simulink model "HEVPlant_Ptbs_V1b_MkSfunc"  (R2018b)
settings: configuration reference "Config_Plant_MkSfunc_FIxStep" (kept outside this file)
PreLoadFcn:
  | HEVPlant_Ptbs_V1_BusInfo
model workspace (MAT data in the model file):
  DiffRatio = 3.421
  EV_current = 200
  EV_motion = [20 4 0.8]
  EV_sf = 2000
  EngDriveRatio = 0.813008130081
  Fs = 0
  Fv = 0.0025
  Jcomp = 0.0227
  Jengine = 0.22
  Ki = 251.3274
  Kisa = 346.6583
  Kp_d = 0.47149
  Kp_q = 0.52125
  Ksa = 85.4316
  Ksf = 1996.2651
  Ld = 0.0003752
  Ldq = [0.0003752 0.0004148]
  Lq = 0.0004148
  Mechanical = [0.0227 0.0025 0]
  MotGbRatio = 1
  P = 4
  PolePairs = 4
  RWheel = 0.3
  Rs = 0.2
  T_max = 120
  T_mtpa = [0 13.3131834767 26.6278836885 39.9456159322 53.2678926341 66.5962219318 79.9321062746 93.277041051 106.632513247 120.000000141]
  b_axle = Simulink.Parameter
  b_axle.Value = 10
  b_axle.DataType = 'auto'
  b_axle.Dimensions = [1 1]
  b_driveshaft = Simulink.Parameter
  b_driveshaft.Value = 10
  b_driveshaft.DataType = 'auto'
  b_driveshaft.Dimensions = [1 1]
  ba = 3.4029
  id_mtpa = [0 -0.114523352646 -0.457989076459 -1.03008464374 -1.83029075221 -2.85788367342 -4.11193850568 -5.59133329791 -7.29475400168 -9.22070020138]
  idq0 = [0 0]
  idq_limits = [-9.220699542 166.993501392 167.247872355]
  iq_mtpa = [0 18.5827440345 37.1633719111 55.7397734896 74.3098506185 92.871523015 111.422734008 129.961456105 148.485696337 166.993501356]
  k_axle = Simulink.Parameter
  k_axle.Value = 5000
  k_axle.DataType = 'auto'
  k_axle.Dimensions = [1 1]
  k_driveshaft = Simulink.Parameter
  k_driveshaft.Value = 1000
  k_driveshaft.DataType = 'auto'
  k_driveshaft.Dimensions = [1 1]
  lambda_pm = 0.1194
  mechanical = [0.0227 0.0025 0]
  mot.max_trq = 307
  mot.max_pwr = 124
  mot.spd = [0 500 1000 1500 2000 2500 3000 3500 3857.04487493 4000 4500 5000 5500 6000 6500 7000 7500 8000 8500 9000 9500 10000 10500 11000 11500 12000 12500]
  mot.trq = [307 307 307 307 307 307 307 307 307 296.028194151 263.136172579 236.822555321 215.29323211 197.352129434 182.171196401 169.158968086 157.881703547 148.014097075 139.307385483 131.568086289 124.643450169 118.41127766 112.772645391 107.646616055 102.9663284 98.676064717 94.7290221283]
  mot.trq_cp = [296.028194151 263.136172579 236.822555321 215.29323211 197.352129434 182.171196401 169.158968086 157.881703547 148.014097075 139.307385483 131.568086289 124.643450169 118.41127766 112.772645391 107.646616055 102.9663284 98.676064717 94.7290221283]
  mot.J = 0.02
  mot.damp = 0.0001
  mot.Tc = 0.0267
  mot.map.spdindex = [0 1000 2000 3000 3857 4000 5000 6000 7000 8000 9000 10000 11000 12000 12584]
  mot.map.trqindex = [10 25 50 75 100 125 150 175 200 225 250 275 300 307]
  mot.map.eff = [84  90  90  90  90  90  90  90  90  90  90  90  90  90  90; 84  90  93  95  95  95  96  95  95  95  95  93  93  93  93; 84  90  93  95  95  95  96  95  96  95  95  95  95  93  93; 84  90  93  95  95  95  96  96  96  95  95  95  95  93  93; 84  90  93  95  95  95  96  96  96  95  95  93  93  93  90; 84  88  90  93  93  95  95  96  95  95  95  93  93  93  90; 84  88  90  90  90  93  95  95  95  93  93  93  93  93  90; 84  88  90  90  90  90  93  93  93  93  93  93  93  93  90; 84  84  88  90  90  90  93  93  93  93  93  93  93  93  90; 84  84  88  90  90  90  90  93  93  93  93  93  93  93  90; 84  84  84  90  90  90  90  93  93  93  93  93  93  93  90; 84  84  84  88  90  90  90  93  93  93  93  93  93  93  90; 84  84  84  88  88  88  90  93  93  93  93  93  93  93  90; 84  84  84  88  88  88  90  93  93  93  93  93  93  93  90]
  mot.m = 30
  mot.Cp = 200
  omega_init = 0
  theta_init = 0
  wc_shaft = Simulink.Parameter
  wc_shaft.Value = 0.1
  wc_shaft.DataType = 'auto'
  wc_shaft.Dimensions = [1 1]
libraries: autolibshared x4, autolibsharedcoupling x2, autolibtransamt x1, autolibshareddiff x1, autolibsharedmappedengines x1, simulink x1, autolibdatasheetbattery x1, autolibmappedmotor x1
(part 1 of 5)
settings Model: Creator=IAEC Nishito  LastModifiedBy=E00026
settings ConfigSetRef: SourceLocation=Base Workspace

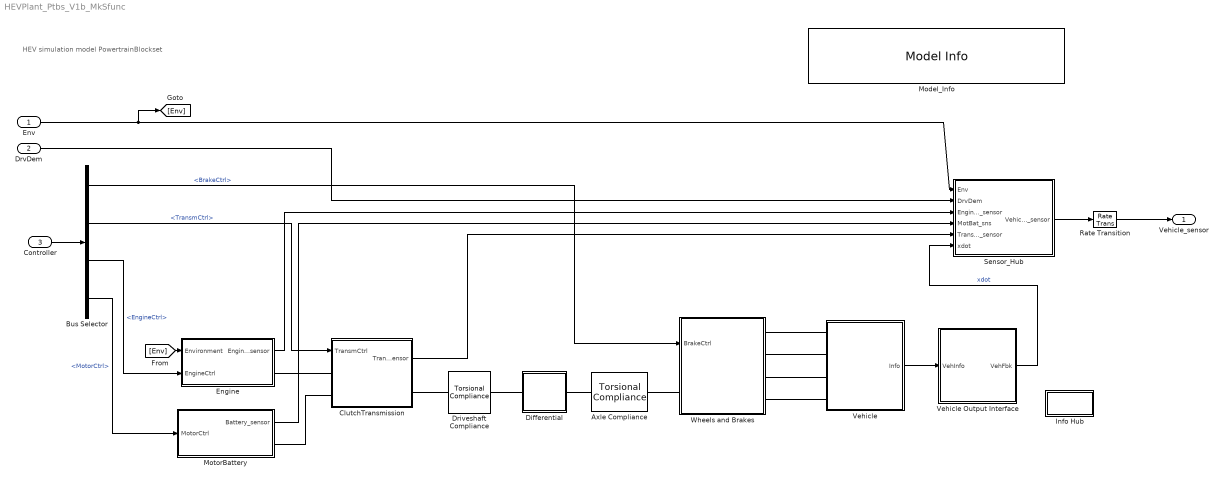
== system HEVPlant_Ptbs_V1b_MkSfunc ==
  note: HEV simulation model
      | PowertrainBlockset
  Env : Inport  OutDataTypeStr=Bus: Environment_Bus  SampleTime=0.001
  DrvDem : Inport  Port=2  OutDataTypeStr=Bus: Driver_demand_Bus  SampleTime=0.001
  Controller : Inport  Port=3  OutDataTypeStr=Bus: Ctrl_intg_Bus  SampleTime=0.001
      settings: AttributesFormatString=%<OutDataTypeStr>
  Axle Compliance : autolibsharedcoupling/Torsional Compliance  port_config=Two-way connection  k=k_axle  b=b_axle  theta_o=0  domega_o=0  omega_c=wc_shaft  blkID=0  aMode=1
      settings: SourceProductName=Powertrain Blockset  SourceProductBaseCode=PW
  Bus Selector : BusSelector  OutputSignals=BrakeCtrl,TransmCtrl,EngineCtrl,MotorCtrl
  ClutchTransmission : Subsystem
  Differential : Subsystem
  Driveshaft Compliance : autolibsharedcoupling/Torsional Compliance  port_config=Two-way connection  k=k_driveshaft  b=b_driveshaft  theta_o=0  domega_o=0  omega_c=wc_shaft  blkID=0  aMode=1
      settings: SourceProductName=Powertrain Blockset  SourceProductBaseCode=PW
  Engine : Subsystem
  Info Hub : Subsystem
  Model_Info : simulink/Model-Wide Utilities/Model Info  Frame=on  DisplayStringWithTags=|  HorizontalTextAlignment=Left  LeftAlignmentValue=0.02
      | Version  %<ModelVersion>
      | LastModifided by %<LastModifiedBy>  Date %<LastModificationDate>
      | Description  %<Description>
  MotorBattery : Subsystem
  Rate Transition : RateTransition  Deterministic=off
  Sensor_Hub : Subsystem
  Vehicle : Subsystem
  Vehicle Output Interface : Subsystem
  Wheels and Brakes : Subsystem
  Vehicle_sensor : Outport  OutDataTypeStr=Bus: Vehicle_sensor_Bus
      settings: AttributesFormatString=%<OutDataTypeStr>
  wires:
  Sensor_Hub/1(Vehicle_sensor) -> Rate Transition/1
  MotorBattery/1(Battery_sensor) -> Sensor_Hub/4(MotBat_sns)
  Env/1 -> [Env], Sensor_Hub/1(Env)
  Bus Selector/3 -> Engine/2(EngineCtrl)  "<EngineCtrl>"
  Bus Selector/1 -> Wheels and Brakes/1(BrakeCtrl)  "<BrakeCtrl>"
  [Env] -> Engine/1(Environment)
  Engine/1(Engine_sensor) -> Sensor_Hub/3(Engine_sensor)
  DrvDem/1 -> Sensor_Hub/2(DrvDem)
  Bus Selector/4 -> MotorBattery/1(MotorCtrl)  "<MotorCtrl>"
  Vehicle Output Interface/1(VehFbk) -> Sensor_Hub/6(xdot)  "xdot"
  Vehicle/1(Info) -> Vehicle Output Interface/1(VehInfo)
  Controller/1 -> Bus Selector/1
  ClutchTransmission/1(Transm_sensor) -> Sensor_Hub/5(Transm_sensor)
  Bus Selector/2 -> ClutchTransmission/1(TransmCtrl)  "<TransmCtrl>"
  Rate Transition/1 -> Vehicle_sensor/1
  connections:
  Driveshaft Compliance/RConn1 -- Differential/LConn1
  Driveshaft Compliance/LConn1 -- ClutchTransmission/RConn1
  Engine/RConn1 -- ClutchTransmission/LConn1
  Wheels and Brakes/RConn2 -- Vehicle/LConn2
  Axle Compliance/LConn1 -- Differential/RConn1
  MotorBattery/RConn1 -- ClutchTransmission/LConn2
  Vehicle/LConn1 -- Wheels and Brakes/RConn1
  Wheels and Brakes/RConn3 -- Vehicle/LConn3
  Axle Compliance/RConn1 -- Wheels and Brakes/LConn1
  Wheels and Brakes/RConn4 -- Vehicle/LConn4

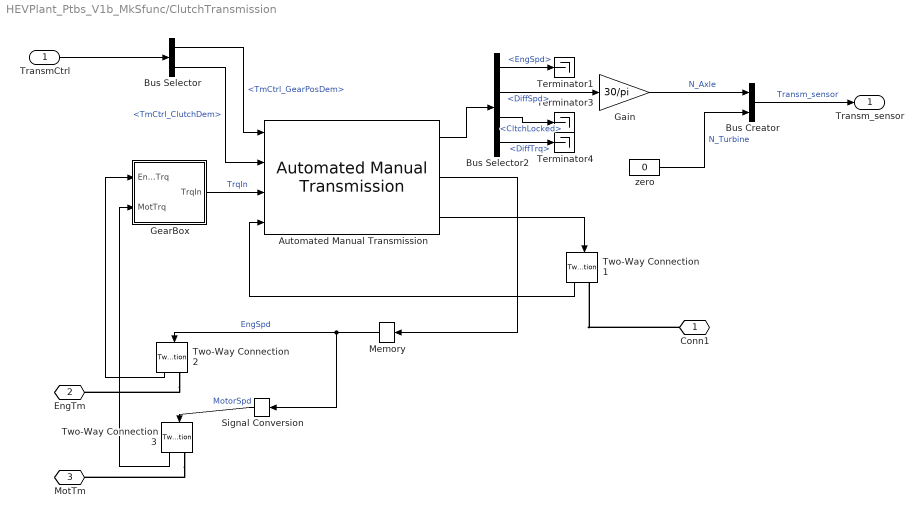
== system HEVPlant_Ptbs_V1b_MkSfunc/ClutchTransmission ==
  TransmCtrl : Inport
  Automated Manual Transmission : autolibtransamt/Automated Manual Transmission  VariantControl=0  cntrlType=External control  TransEffModelPopup=Gear only  Jin=.3  bin=.03  omegain_o=0  G=[-1, 0, 1, 2, 3, 4, 5]  Trq_bpts=[25, 50, 75, 100, 150, 200, 250]  omega_bpts=[52.4 78.5 105 131 157 183 209 262 314 419 524]  Temp_bpts=[313 358]  N=[-4.47 ,1, 4.47, 2.47, 1.47, 1, 0.8]  Jout=[0.128 0.01 0.128 0.1 0.062 0.028 0.01]  bout=[.003 .001 .003 .0025 .002 .001 .001]  eta=[0.9, 0.9, 0.9, 0.9, 0.9, 0.95, 0.95]  eta_tbl=reshape([0.53 0.71 0.77 0.79 0.82 0.82 0.82 0.5 0.7 0.77 0.79 0.82 0.82 0.82 0.54 0.72 0.78 0.81 0.83 0.82 0.82 0.56 0.73 0.79 0.81 0.84 0.82 0.82 0.58 0.74 0.79 0.82 0.84 0.82 0.82 0.57 0.74 0.79 0.82 0.84 0.82 0.82 0.58 0.74 0.79 0.82 0.84 0.82 0.82 0.58 0.74 0.79 0.82 0.84 0.82 0.82 0.57 0.74 0.8 0.82 0.85 0.82 0.82 0.55 0.73 0.78 0.81 0.84 0.82 0.82 0.51 0.71 0.77 0.81 0.84 0.82 0.82 0.53 0.71 0.77 0.79 0.82 0.82 0.82 0.5 0.7 0.77 0.79 0.82 0.82 0.82 0.54 0.72 0.78 0.81 0.83 0.82 0.82 0.56 0.73 0.79 0.81 0.84 0.82 0.82 0.58 0.74 0.79 0.82 0.84 0.82 0.82 0.57 0.74 0.79 0.82 0.84 0.82 0.82 0.58 0.74 0.79 0.82 0.84 0.82 0.82 0.58 0.74 0.79 0.82 0.84 0.82 0.82 0.57 0.74 0.8 0.82 0.85 0.82 0.82 0.55 0.73 0.78 0.81 0.84 0.82 0.82 0.51 0.71 0.77 0.81 0.84 0.82 0.82 0.53 0.71 0.77 0.79 0.82 0.82 0.82 0.5 0.7 0.77 0.79 0.82 0.82 0.82 0.54 0.72 0.78 0.81 0.83 0.82 0.82 0.56 0.73 0.79 0.81 0.84 0.82 0.82 0.58 0.74 0.79 0.82 0.84 0.82 0.82 0.57 0.74 0.79 0.82 0.84 0.82 0.82 0.58 0.74 0.79 0.82 0.84 0.82 0.82 0.58 0.74 0.79 0.82 0.84 0.82 0.82 0.57 0.74 0.8 0.82 0.85 0.82 0.82 0.55 0.73 0.78 0.81 0.84 0.82 0.82 0.51 0.71 0.77 0.81 0.84 0.82 0.82 0.7 0.79 0.82 0.83 0.84 0.84 0.84 0.63 0.76 0.8 0.82 0.83 0.84 0.84 0.58 0.74 0.79 0.81 0.83 0.84 0.84 0.58 0.74 0.79 0.81 0.83 0.84 0.84 0.58 0.74 0.79 0.81 0.84 0.84 0.84 0.57 0.73 0.78 0.81 0.84 0.85 0.84 0.57 0.73 0.79 0.81 0.84 0.85 0.84 0.56 0.73 0.78 0.81 0.83 0.85 0.84 0.55 0.73 0.78 0.81 0.84 0.85 0.84 0.52 0.71 0.77 0.8 0.83 0.85 0.84 0.48 0.69 0.76 0.79 0.83 0.84 0.84 0.64 0.76 0.8 0.81 0.83 0.84 0.84 0.56 0.73 0.78 0.8 0.83 0.84 0.84 0.54 0.71 0.77 0.8 0.82 0.84 0.84 0.53 0.71 0.77 0.8 0.83 0.84 0.84 0.51 0.71 0.77 0.8 0.83 0.84 0.85 0.52 0.7 0.77 0.8 0.83 0.84 0.85 0.51 0.71 0.76 0.79 0.83 0.84 0.85 0.5 0.69 0.76 0.79 0.82 0.84 0.85 0.45 0.68 0.75 0.78 0.82 0.84 0.85 0.43 0.67 0.74 0.78 0.81 0.83 0.84 0.38 0.63 0.71 0.75 0.8 0.82 0.83 0.65 0.79 0.84 0.85 0.88 0.89 0.89 0.56 0.75 0.81 0.83 0.86 0.88 0.89 0.52 0.72 0.79 0.83 0.86 0.88 0.88 0.51 0.72 0.79 0.83 0.86 0.88 0.89 0.49 0.71 0.78 0.82 0.86 0.88 0.89 0.47 0.7 0.78 0.82 0.86 0.87 0.88 0.45 0.69 0.77 0.81 0.85 0.87 0.88 0.4 0.67 0.75 0.8 0.84 0.86 0.88 0.3 0.64 0.73 0.78 0.83 0.86 0.87 0.17 0.55 0.67 0.73 0.8 0.83 0.85 0.089 0.45 0.61 0.69 0.77 0.81 0.83 0.61 0.75 0.82 0.84 0.87 0.87 0.88 0.54 0.73 0.8 0.82 0.86 0.87 0.88 0.51 0.71 0.79 0.82 0.86 0.87 0.88 0.52 0.72 0.79 0.82 0.86 0.87 0.89 0.52 0.72 0.8 0.83 0.86 0.88 0.89 0.53 0.72 0.79 0.82 0.86 0.87 0.89 0.5 0.7 0.78 0.82 0.86 0.88 0.88 0.46 0.69 0.77 0.81 0.85 0.87 0.88 0.4 0.67 0.75 0.8 0.83 0.86 0.88 0.33 0.64 0.73 0.78 0.83 0.85 0.87 0.33 0.64 0.73 0.78 0.83 0.85 0.87 0.78 0.85 0.87 0.88 0.89 0.89 0.89 0.73 0.83 0.86 0.88 0.89 0.89 0.89 0.72 0.83 0.86 0.88 0.89 0.89 0.89 0.72 0.83 0.87 0.89 0.9 0.89 0.89 0.72 0.83 0.87 0.88 0.9 0.89 0.89 0.71 0.83 0.87 0.88 0.9 0.89 0.89 0.71 0.83 0.86 0.88 0.9 0.89 0.89 0.7 0.82 0.86 0.88 0.9 0.89 0.89 0.69 0.82 0.86 0.88 0.9 0.89 0.89 0.67 0.81 0.86 0.88 0.9 0.89 0.89 0.63 0.79 0.85 0.87 0.89 0.89 0.89 0.78 0.85 0.87 0.88 0.89 0.89 0.89 0.73 0.83 0.86 0.88 0.89 0.89 0.89 0.72 0.83 0.86 0.88 0.89 0.89 0.89 0.72 0.83 0.87 0.89 0.9 0.89 0.89 0.72 0.83 0.87 0.88 0.9 0.89 0.89 0.71 0.83 0.87 0.88 0.9 0.89 0.89 0.71 0.83 0.86 0.88 0.9 0.89 0.89 0.7 0.82 0.86 0.88 0.9 0.89 0.89 0.69 0.82 0.86 0.88 0.9 0.89 0.89 0.67 0.81 0.86 0.88 0.9 0.89 0.89 0.63 0.79 0.85 0.87 0.89 0.89 0.89 0.78 0.85 0.87 0.88 0.89 0.89 0.89 0.73 0.83 0.86 0.88 0.89 0.89 0.89 0.72 0.83 0.86 0.88 0.89 0.89 0.89 0.72 0.83 0.87 0.89 0.9 0.89 0.89 0.72 0.83 0.87 0.88 0.9 0.89 0.89 0.71 0.83 0.87 0.88 0.9 0.89 0.89 0.71 0.83 0.86 0.88 0.9 0.89 0.89 0.7 0.82 0.86 0.88 0.9 0.89 0.89 0.69 0.82 0.86 0.88 0.9 0.89 0.89 0.67 0.81 0.86 0.88 0.9 0.89 0.89 0.63 0.79 0.85 0.87 0.89 0.89 0.89 0.82 0.87 0.88 0.89 0.89 0.89 0.89 0.81 0.87 0.89 0.89 0.9 0.9 0.89 0.76 0.85 0.87 0.89 0.9 0.89 0.89 0.72 0.83 0.86 0.88 0.89 0.89 0.89 0.72 0.83 0.86 0.88 0.89 0.9 0.89 0.71 0.82 0.86 0.88 0.89 0.9 ...(+1314 chars))  omegaout_o=0  G_o=0  tauc=.02  ts=.15  tc=0.25  R=.2  K_c=5e3  mus=0.6  muk=0.4  ClutchLocked=off  SynchLocked=off  maxAbsSpd=5e3
      settings: SourceProductName=Powertrain Blockset  SourceProductBaseCode=PW
  Bus Creator : BusCreator  Inputs=2  OutDataTypeStr=Bus: Transm_sensor_Bus
      settings: AttributesFormatString=%<OutDataTypeStr>
  Bus Selector : BusSelector  OutputSignals=TmCtrl_GearPosDem,TmCtrl_ClutchDem
  Bus Selector2 : BusSelector  OutputSignals=Eng.EngSpd,Diff.DiffSpd,Cltch.CltchLocked,Diff.DiffTrq
  Gain : Gain  Gain=30/pi
  GearBox : Subsystem
  Memory : Memory
  Signal Conversion : SignalConversion  OverrideOpt=off
  Terminator1 : Terminator
  Terminator3 : Terminator
  Terminator4 : Terminator
  Two-Way Connection1 : TwoWayConnection
  Two-Way Connection2 : TwoWayConnection
  Two-Way Connection3 : TwoWayConnection
  zero : Constant  Value=0
  Conn1 : PMIOPort  Side=Right
  EngTm : PMIOPort  Port=2  Side=Left
  MotTm : PMIOPort  Port=3  Side=Left
  Transm_sensor : Outport
  wires:
  TransmCtrl/1 -> Bus Selector/1
  Automated Manual Transmission/2 -> Memory/1
  Automated Manual Transmission/1 -> Bus Selector2/1
  Bus Selector2/3 -> Terminator3/1  "<CltchLocked>"
  Automated Manual Transmission/3 -> Two-Way Connection1/1
  GearBox/1(TrqIn) -> Automated Manual Transmission/3  "TrqIn"
  Two-Way Connection1/1 -> Automated Manual Transmission/4
  Bus Selector2/4 -> Terminator4/1  "<DiffTrq>"
  Two-Way Connection3/1 -> GearBox/2(MotTrq)
  Two-Way Connection2/1 -> GearBox/1(EngineTrq)
  Memory/1 -> Two-Way Connection2/1, Signal Conversion/1  "EngSpd"
  Bus Selector2/1 -> Terminator1/1  "<EngSpd>"
  Gain/1 -> Bus Creator/1  "N_Axle"
  Bus Selector2/2 -> Gain/1  "<DiffSpd>"
  zero/1 -> Bus Creator/2  "N_Turbine"
  Bus Creator/1 -> Transm_sensor/1  "Transm_sensor"
  Bus Selector/1 -> Automated Manual Transmission/1  "<TmCtrl_GearPosDem>"
  Bus Selector/2 -> Automated Manual Transmission/2  "<TmCtrl_ClutchDem>"
  Signal Conversion/1 -> Two-Way Connection3/1  "MotorSpd"
  connections:
  Conn1/RConn1 -- Two-Way Connection1/RConn1
  Two-Way Connection2/RConn1 -- EngTm/RConn1
  Two-Way Connection3/RConn1 -- MotTm/RConn1

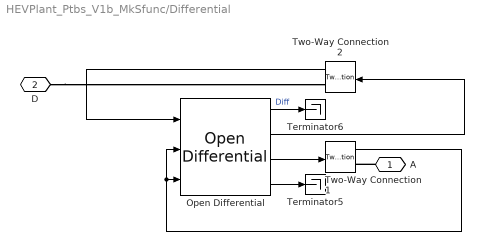
== system HEVPlant_Ptbs_V1b_MkSfunc/Differential ==
  Open Differential : autolibshareddiff/Open Differential  shaftSwitchMask=To the left of center-line  Ndiff=DiffRatio  Jd=.025  bd=1e-3  Jw1=.01  bw1=1e-3  Jw2=.01  bw2=1e-3  omegaw1o=0  omegaw2o=0  maxAbsSpd=5e3  aMode=1
      settings: SourceProductName=Powertrain Blockset  SourceProductBaseCode=PW
  Terminator5 : Terminator
  Terminator6 : Terminator
  Two-Way Connection1 : TwoWayConnection
  Two-Way Connection2 : TwoWayConnection
  A : PMIOPort  Side=Right
  D : PMIOPort  Port=2  Side=Left
  wires:
  Open Differential/3 -> Two-Way Connection1/1
  Open Differential/4 -> Terminator5/1
  Open Differential/1 -> Terminator6/1  "Diff"
  Open Differential/2 -> Two-Way Connection2/1
  Two-Way Connection1/1 -> Open Differential/2, Open Differential/3
  Two-Way Connection2/1 -> Open Differential/1
  connections:
  A/RConn1 -- Two-Way Connection1/RConn1
  D/RConn1 -- Two-Way Connection2/RConn1

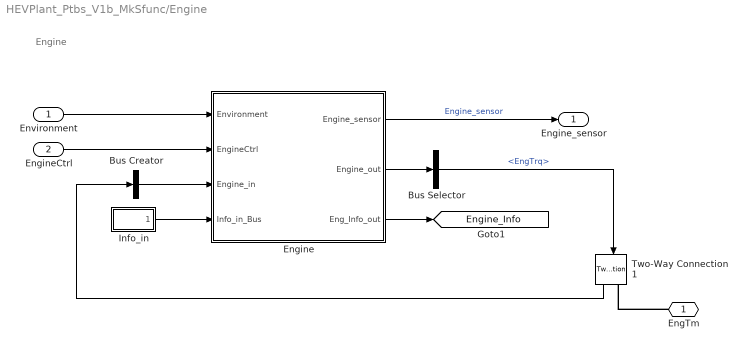
== system HEVPlant_Ptbs_V1b_MkSfunc/Engine ==
  note: Engine
  Environment : Inport
  EngineCtrl : Inport  Port=2
  Bus Creator : BusCreator  Inputs=1
  Bus Selector : BusSelector  OutputSignals=EngTrq
  Engine : Subsystem
  Info_in : Subsystem
  Two-Way Connection1 : TwoWayConnection
  EngTm : PMIOPort  Side=Right
  Engine_sensor : Outport
  tag scope: Engine_Info=global
  wires:
  Two-Way Connection1/1 -> Bus Creator/1
  Bus Selector/1 -> Two-Way Connection1/1  "<EngTrq>"
  Environment/1 -> Engine/1(Environment)
  EngineCtrl/1 -> Engine/2(EngineCtrl)
  Bus Creator/1 -> Engine/3(Engine_in)
  Info_in/1(Info_in) -> Engine/4(Info_in_Bus)
  Engine/1(Engine_sensor) -> Engine_sensor/1  "Engine_sensor"
  Engine/2(Engine_out) -> Bus Selector/1
  Engine/3(Eng_Info_out) -> [Engine_Info]
  connections:
  EngTm/RConn1 -- Two-Way Connection1/RConn1

== system HEVPlant_Ptbs_V1b_MkSfunc/Info Hub ==
  Terminator1 : Terminator
  wires:
  [Engine_Info] -> Terminator1/1

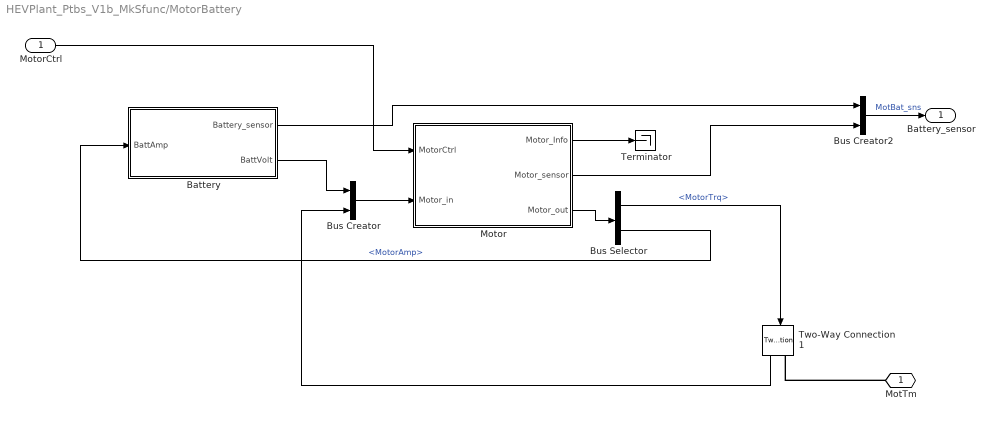
== system HEVPlant_Ptbs_V1b_MkSfunc/MotorBattery ==
  MotorCtrl : Inport
  Battery : Subsystem  TreatAsAtomicUnit=on
  Bus Creator : BusCreator  Inputs=2
  Bus Creator2 : BusCreator  Inputs=2
  Bus Selector : BusSelector  OutputSignals=MotorTrq,MotorAmp
  Motor : Subsystem
  Terminator : Terminator
  Two-Way Connection1 : TwoWayConnection
  MotTm : PMIOPort  Side=Right
  Battery_sensor : Outport
  wires:
  Bus Creator2/1 -> Battery_sensor/1  "MotBat_sns"
  MotorCtrl/1 -> Motor/1(MotorCtrl)
  Two-Way Connection1/1 -> Bus Creator/2
  Motor/2(Motor_sensor) -> Bus Creator2/2
  Battery/1(Battery_sensor) -> Bus Creator2/1
  Battery/2(BattVolt) -> Bus Creator/1
  Motor/3(Motor_out) -> Bus Selector/1
  Bus Selector/1 -> Two-Way Connection1/1  "<MotorTrq>"
  Bus Selector/2 -> Battery/1(BattAmp)  "<MotorAmp>"
  Motor/1(Motor_Info) -> Terminator/1
  Bus Creator/1 -> Motor/2(Motor_in)
  connections:
  MotTm/RConn1 -- Two-Way Connection1/RConn1

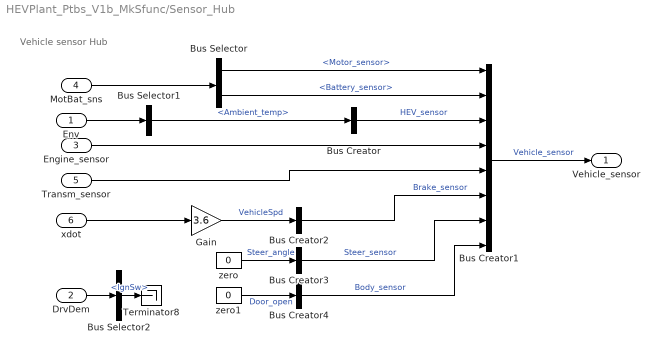
== system HEVPlant_Ptbs_V1b_MkSfunc/Sensor_Hub ==
  note: Vehicle sensor Hub
  Env : Inport
  DrvDem : Inport  Port=2
  Engine_sensor : Inport  Port=3
  MotBat_sns : Inport  Port=4
  Transm_sensor : Inport  Port=5
  xdot : Inport  Port=6
  Bus Creator : BusCreator  Inputs=1  OutDataTypeStr=Bus: HEV_sensor_Bus
      settings: AttributesFormatString=%<OutDataTypeStr>
  Bus Creator1 : BusCreator  Inputs=8  OutDataTypeStr=Bus:Vehicle_sensor_Bus
      settings: AttributesFormatString=%<OutDataTypeStr>
  Bus Creator2 : BusCreator  Inputs=1  OutDataTypeStr=Bus: Brake_sensor_Bus
      settings: AttributesFormatString=%<OutDataTypeStr>
  Bus Creator3 : BusCreator  Inputs=1  OutDataTypeStr=Bus: Steer_sensor_Bus
      settings: AttributesFormatString=%<OutDataTypeStr>
  Bus Creator4 : BusCreator  Inputs=1  OutDataTypeStr=Bus: Body_sensor_Bus
      settings: AttributesFormatString=%<OutDataTypeStr>
  Bus Selector : BusSelector  OutputSignals=Motor_sensor,Battery_sensor
  Bus Selector1 : BusSelector  OutputSignals=Ambient_temp
  Bus Selector2 : BusSelector  OutputSignals=IgnSw
  Gain : Gain  Gain=3.6
  Terminator8 : Terminator
  zero : Constant  Value=0
  zero1 : Constant  Value=0
  Vehicle_sensor : Outport
      settings: AttributesFormatString=%<OutDataTypeStr>
  wires:
  Bus Creator1/1 -> Vehicle_sensor/1  "Vehicle_sensor"
  Engine_sensor/1 -> Bus Creator1/4
  xdot/1 -> Gain/1
  MotBat_sns/1 -> Bus Selector/1
  Bus Selector/1 -> Bus Creator1/1  "<Motor_sensor>"
  Bus Selector/2 -> Bus Creator1/2  "<Battery_sensor>"
  Bus Creator/1 -> Bus Creator1/3  "HEV_sensor"
  Transm_sensor/1 -> Bus Creator1/5
  Gain/1 -> Bus Creator2/1  "VehicleSpd"
  Bus Creator2/1 -> Bus Creator1/6  "Brake_sensor"
  zero/1 -> Bus Creator3/1  "Steer_angle"
  zero1/1 -> Bus Creator4/1  "Door_open"
  Bus Creator3/1 -> Bus Creator1/7  "Steer_sensor"
  Bus Creator4/1 -> Bus Creator1/8  "Body_sensor"
  DrvDem/1 -> Bus Selector2/1
  Env/1 -> Bus Selector1/1
  Bus Selector1/1 -> Bus Creator/1  "<Ambient_temp>"
  Bus Selector2/1 -> Terminator8/1  "<IgnSw>"

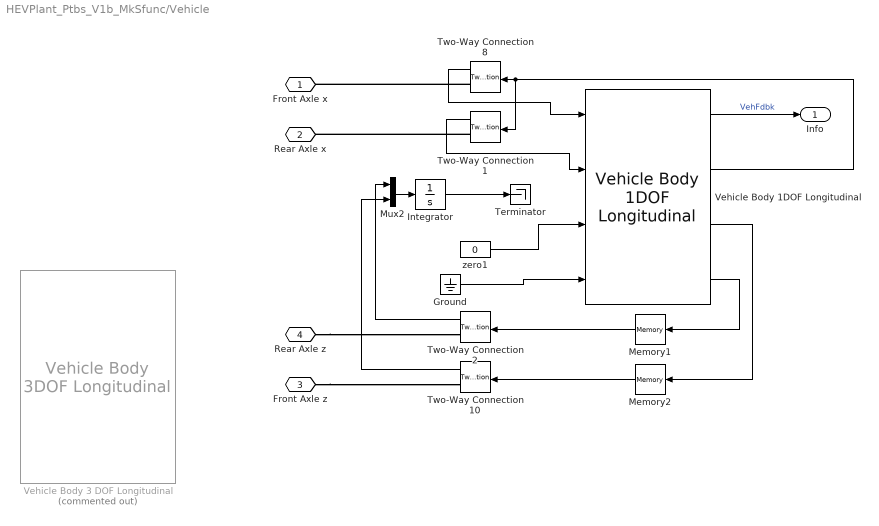
== system HEVPlant_Ptbs_V1b_MkSfunc/Vehicle ==
  Ground : Ground
  Integrator : Integrator
  Memory1 : Memory
  Memory2 : Memory
  Mux2 : Mux  Inputs=2
  Terminator : Terminator
  Two-Way Connection{1..2,8,10} (4 alike) : TwoWayConnection
  Vehicle Body 1DOF Longitudinal : autolibshared/Vehicle Body 1DOF Longitudinal  VariantControl=SL  aMode=1  NF=2  NR=2  m=1.723200000000000e+03  a=1.56  b=1.22  h=.5  Cd=.29  Af=2.27  x_o=0  xdot_o=0  Pabs=101325  T=273  g=9.81
      settings: SourceProductName=Powertrain Blockset  SourceProductBaseCode=PW
  Vehicle Body 3 DOF Longitudinal : autolibshared/Vehicle Body 3DOF Longitudinal  Commented=on  VariantControl=SL  groundType=Axle displacement, velocity  aMode=aMode  NF=2  NR=2  m=1.723200000000000e+03  a=1.56  b=1.22  h=.5  Cd=.29  Af=2.27  x_o=0  xdot_o=0  Cl=.1  z_o=-.35  zdot_o=0  Iyy=3000  Cpm=.1  theta_o=0  q_o=0  FskF=[-50, -1, 0, 2, 3, 52].*1.25e4  dzsF=[-5e-3, -1e-4, 0, .2, .2001, .2051]  FsbF=[-10000 -100 -10 0 10 100 10000]  dzdotsF=[-10 -1 -.1 0 .1 1 10]  FskR=[-50, -1, 0, 2, 3, 52].*7.5e3  dzsR=[-5e-3, -1e-4, 0, .2, .2001, .2051]  FsbR=[-10000 -100 -10 0 10 100 10000]  dzdotsR=[-10 -1 -.1 0 .1 1 10]  Pabs=101325  T=273  g=9.81  blkID=0
      settings: SourceProductName=Powertrain Blockset  SourceProductBaseCode=PW
  zero1 : Constant  Value=0
  Front Axle x : PMIOPort  Side=Left
  Rear Axle x : PMIOPort  Port=2  Side=Left
  Front Axle z : PMIOPort  Port=3  Side=Left
  Rear Axle z : PMIOPort  Port=4  Side=Left
  Info : Outport
  wires:
  Vehicle Body 1DOF Longitudinal/3 -> Memory2/1
  Two-Way Connection8/1 -> Vehicle Body 1DOF Longitudinal/1
  Vehicle Body 1DOF Longitudinal/1 -> Info/1  "VehFdbk"
  Ground/1 -> Vehicle Body 1DOF Longitudinal/4
  Two-Way Connection1/1 -> Vehicle Body 1DOF Longitudinal/2
  Vehicle Body 1DOF Longitudinal/4 -> Memory1/1
  Two-Way Connection2/1 -> Mux2/1
  Two-Way Connection10/1 -> Mux2/2
  Mux2/1 -> Integrator/1
  Integrator/1 -> Terminator/1
  zero1/1 -> Vehicle Body 1DOF Longitudinal/3
  Vehicle Body 1DOF Longitudinal/2 -> Two-Way Connection1/1, Two-Way Connection8/1
  Memory1/1 -> Two-Way Connection2/1
  Memory2/1 -> Two-Way Connection10/1
  connections:
  Two-Way Connection8/RConn1 -- Front Axle x/RConn1
  Front Axle z/RConn1 -- Two-Way Connection10/RConn1
  Two-Way Connection1/RConn1 -- Rear Axle x/RConn1
  Rear Axle z/RConn1 -- Two-Way Connection2/RConn1

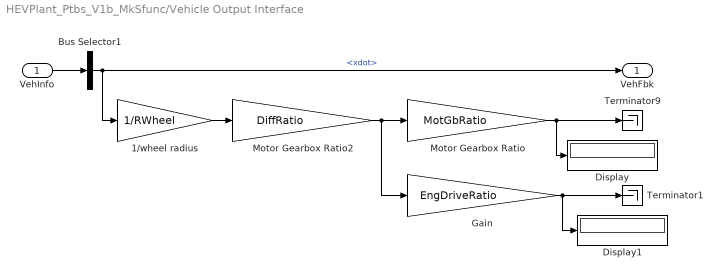
== system HEVPlant_Ptbs_V1b_MkSfunc/Vehicle Output Interface ==
  VehInfo : Inport
  1/wheel radius : Gain  Gain=1/RWheel
  Bus Selector1 : BusSelector  OutputSignals=BdyFrm.Cg.Vel.xdot
  Display : Display
  Display1 : Display
  Gain : Gain  Gain=EngDriveRatio
  Motor Gearbox Ratio : Gain  Gain=MotGbRatio
  Motor Gearbox Ratio2 : Gain  Gain=DiffRatio
  Terminator1 : Terminator
  Terminator9 : Terminator
  VehFbk : Outport
  wires:
  Bus Selector1/1 -> VehFbk/1, 1/wheel radius/1  "<xdot>"
  Gain/1 -> Display1/1, Terminator1/1
  Motor Gearbox Ratio/1 -> Display/1, Terminator9/1
  VehInfo/1 -> Bus Selector1/1
  Motor Gearbox Ratio2/1 -> Gain/1, Motor Gearbox Ratio/1
  1/wheel radius/1 -> Motor Gearbox Ratio2/1
